simulink model "linear_system"  (R2024b)
settings: Solver=VariableStepAuto  StartTime=0.0  StopTime=10  RelTol=1e-3
values from neighbouring files (symbols this model uses):
  A = double(A_matrix)    [Modelling_AB_Matrix_Calculation.m]
  B = double(B_matrix)    [Modelling_AB_Matrix_Calculation.m]
  C = eye(size(A))    [Modelling_AB_Matrix_Calculation.m]
  config = [l_f, l_r, l_b, l_l]    [Modelling_AB_Matrix_Calculation.m]    (also in Non_linear_trim_solver.m = configs(i, :))
  K = [-0.1 2.30105727721e-17 0.1 -1.6517764485e-17 2.5369137881e-16 -0.1 7.90565190817e-17 0.1 0.158113883008 0.158113883008 0.158113883008 0.158113883008 ... (48 elements, 4x12)]    [K_reference.mat]
libraries: uavutilslib x3
settings Model: Creator=kaleb  LastModifiedBy=kaleb

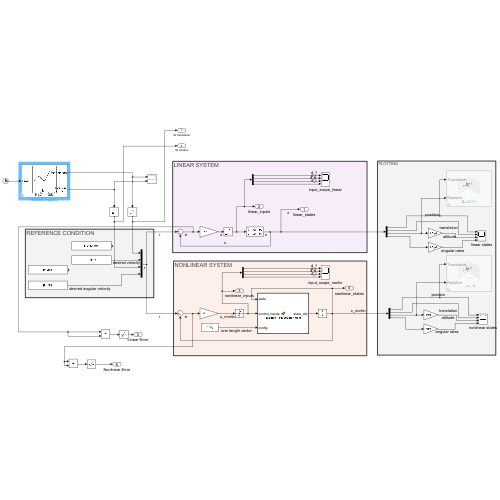
[thumbnail: Simulink's stored preview of the top-level diagram]
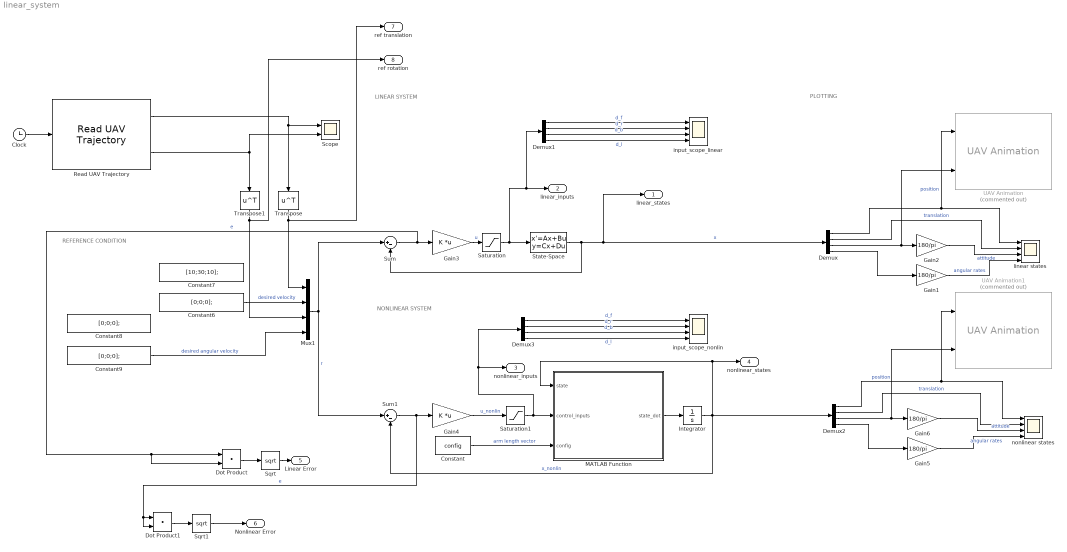
== system linear_system ==
  note: PLOTTING
  note: REFERENCE CONDITION
  note: LINEAR SYSTEM
  note: NONLINEAR SYSTEM
  Clock : Clock
  Constant : Constant  Value=config  OutDataTypeStr=Inherit: Inherit via back propagation
  Constant6 : Constant  Value=[0;0;0];  SampleTime=1/50
  Constant7 : Constant  Value=[10;30;10];  SampleTime=1/50
  Constant8 : Constant  Value=[0;0;0];  SampleTime=1/50
  Constant9 : Constant  Value=[0;0;0];  SampleTime=1/50
  Demux{,1..3} (4 alike) : Demux
  Dot Product : DotProduct  OutDataTypeStr=Inherit: Inherit via internal rule
  Dot Product1 : DotProduct  OutDataTypeStr=Inherit: Inherit via internal rule
  Gain{1..2,5..6} (4 alike) : Gain  Gain=180/pi
  Gain3 : Gain  Gain=K  Multiplication=Matrix(K*u)
  Gain4 : Gain  Gain=K  Multiplication=Matrix(K*u)
  Integrator : Integrator  InitialCondition=[0,0,0 ,5,0,0 ,0,-pi/4,0 ,0,0,0]'
  MATLAB Function : MATLAB Function  TreatAsAtomicUnit=on
  Mux1 : Mux
  Read UAV Trajectory : uavutilslib/Read UAV Trajectory  TrajectorySource=From trajectory object in workspace  ScenarioObj=singleUAVScenario  PlatformName=UAV  TrajectoryObj=T  TransformToENU=off  FrameConversionDisplay=NED → NED
  Saturation : Saturate  UpperLimit=10  LowerLimit=-10
  Saturation1 : Saturate  UpperLimit=20  LowerLimit=-20
  Scope : Scope  NumInputPorts=2
  Sqrt : Sqrt
  Sqrt1 : Sqrt
  State-Space : StateSpace  A=A  B=B  C=C  D=zeros(12,4)  InitialCondition=[0,0,0, 5,0,0, 0,-pi/4,0, 0,0,0];  ContinuousStateAttributes={'pn','pe','h','u','v','w','phi','theta','psi','p','q','r'}
  Sum : Sum  Inputs=|+-
  Sum1 : Sum  Inputs=|+-
  Transpose : Math  Operator=transpose
  Transpose1 : Math  Operator=transpose
  UAV Animation : uavutilslib/UAV Animation  Commented=on  NumUAV=1  DynamicUAVConfig=off  UAVType=Multirotor  UAVSize=0.5  UAVColor=[0.5 0.5 0.5]  UAVTrajectoryAlpha=1  InertialZDirection=Down  RotationFormat=Euler ZYX  DrawMarkers=off  SampleTime=0.1
  UAV Animation1 : uavutilslib/UAV Animation  Commented=on  NumUAV=1  DynamicUAVConfig=off  UAVType=Multirotor  UAVSize=0.5  UAVColor=[0.5 0.5 0.5]  UAVTrajectoryAlpha=1  InertialZDirection=Down  RotationFormat=Euler ZYX  DrawMarkers=off  SampleTime=0.1
  input_scope_linear : Scope  NumInputPorts=4
  input_scope_nonlin : Scope  NumInputPorts=4
  linear states : Scope  NumInputPorts=4
  nonlinear states : Scope  NumInputPorts=4
  linear_states : Outport
  linear_inputs : Outport  Port=2
  nonlinear_inputs : Outport  Port=3
  nonlinear_states : Outport  Port=4
  Linear Error : Outport  Port=5
  Nonlinear Error : Outport  Port=6
  ref translation : Outport  Port=7
  ref rotation : Outport  Port=8
  wires:
  State-Space/1 -> linear_states/1, Demux/1, Sum/2  "x"
  Demux1/1 -> input_scope_linear/1  "d_f"
  Demux1/2 -> input_scope_linear/2  "d_r"
  Demux1/3 -> input_scope_linear/3  "d_b"
  Demux1/4 -> input_scope_linear/4  "d_l"
  Gain3/1 -> Saturation/1  "u"
  Sum/1 -> Gain3/1, Dot Product/1, Dot Product/2  "e"
  Gain4/1 -> Saturation1/1  "u_nonlin"
  Constant/1 -> MATLAB Function/3(config)  "arm length vector"
  Integrator/1 -> Sum1/2, Demux2/1, MATLAB Function/1(state), nonlinear_states/1  "x_nonlin"
  MATLAB Function/1(state_dot) -> Integrator/1
  Sum1/1 -> Gain4/1, Dot Product1/1, Dot Product1/2  "e"
  Demux2/1 -> nonlinear states/1, UAV Animation1/1  "position"
  Demux2/2 -> nonlinear states/2  "translation"
  Demux2/3 -> Gain6/1, UAV Animation1/2
  Demux2/4 -> Gain5/1
  Gain5/1 -> nonlinear states/4  "angular rates"
  Gain6/1 -> nonlinear states/3  "attitude"
  Demux/2 -> linear states/2  "translation"
  Gain2/1 -> linear states/3  "attitude"
  Demux/1 -> linear states/1, UAV Animation/1  "position"
  Gain1/1 -> linear states/4  "angular rates"
  Demux/4 -> Gain1/1
  Demux/3 -> UAV Animation/2, Gain2/1
  Demux3/2 -> input_scope_nonlin/2  "d_r"
  Demux3/3 -> input_scope_nonlin/3  "d_b"
  Demux3/1 -> input_scope_nonlin/1  "d_f"
  Demux3/4 -> input_scope_nonlin/4  "d_l"
  Constant9/1 -> Mux1/4  "desired angular velocity"
  Constant6/1 -> Mux1/2  "desired velocity"
  Mux1/1 -> Sum/1, Sum1/1  "r"
  Sqrt/1 -> Linear Error/1
  Dot Product/1 -> Sqrt/1
  Sqrt1/1 -> Nonlinear Error/1
  Dot Product1/1 -> Sqrt1/1
  Saturation1/1 -> Demux3/1, nonlinear_inputs/1, MATLAB Function/2(control_inputs)
  Saturation/1 -> Demux1/1, linear_inputs/1, State-Space/1
  Clock/1 -> Read UAV Trajectory/1
  Read UAV Trajectory/1 -> Transpose/1, Scope/1
  Read UAV Trajectory/2 -> Scope/2, Transpose1/1
  Transpose/1 -> Mux1/1, ref translation/1
  Transpose1/1 -> ref rotation/1, Mux1/3

== matlab function linear_system/MATLAB Function ==
  data: state input; control_inputs input; config input; state_dot output
%% Equation of motion calculation
function state_dot = calculate_quadcopter_eom(state, control_inputs, config)

l_f = config(1);
l_r = config(2);
l_b = config(3);
l_l = config(4);

% state_dot = zeros(12, 1);

t_motor = 31/1000;   % Motor thickness (m)
t_prop = 2/1000;    % Propeller thickness (m)
d_cube = 0.10;    % Cube dimension (m)
m_motor = 58/1000;   % Motor mass (kg)
m_prop = 21/1000;    % Propeller mass (kg)
m_arm = 65/1000;     % Arm mass (kg)
m_cube = 0.69;    % Cube mass (kg)
r_motor = 28/1000;   % Motor radius (m)
r_prop = 25.4/100;    % Propeller radius (m)

g = 9.81; % Gravity (kg/m^2)
k1 = 1;   % Thrust coefficient
k2 = 0.2; % Torque coefficient

[CG_matrix, J_matrix_body, m_tot] = calculate_CG_Moment_of_inertia(config);

X_cg = CG_matrix(1);
Y_cg = CG_matrix(2);

% Function to calculate the equations of motion of the quadcopter
% Inputs:
%   state: [pn; pe; h; u; v; w; phi; theta; psi; p; q; r]
%   control_inputs: [delta_f; delta_r; delta_b; delta_l]
%   J_matrix_body: Moment of inertia matrix [Jx, Jy, Jz]
%   m_tot: Total mass of the quadcopter
%   k1: Thrust coefficient
%   k2: Torque coefficient
%   g: Gravitational acceleration
%   l_f, l_r, l_b, l_l: Individual arm lengths for front, right, back, and left rotors
% Outputs:
%   state_dot: Time derivatives of the state vector
% load_constant_values

% Extract state variables
pn = state(1); pe = state(2); h = state(3);
u = state(4); v = state(5); w = state(6);
phi = state(7); theta = state(8); psi = state(9);
p = state(10); q = state(11); r = state(12);
% 
% Extract control inputs
delta_f = control_inputs(1);
delta_r = control_inputs(2);
delta_b = control_inputs(3);
delta_l = control_inputs(4);

% Position Dynamics
position_matrix = [
    cos(theta)*cos(psi), sin(phi)*sin(theta)*cos(psi) - cos(phi)*sin(psi), cos(phi)*sin(theta)*cos(psi) + sin(phi)*sin(psi);
    cos(theta)*sin(psi), sin(phi)*sin(theta)*sin(psi) + cos(phi)*cos(psi), cos(phi)*sin(theta)*sin(psi) - sin(phi)*cos(psi);
    sin(theta), -sin(phi)*cos(theta), -cos(phi)*cos(theta)
    ];
position_vector = [u; v; w];
position_dot = position_matrix * position_vector;

% Linear Velocity Dynamics
linear_velocity_matrix = [
    0, r, -q;
    -r, 0, p;
    q, -p, 0
    ];
gravity_vector = [-g*sin(theta); g*cos(theta)*sin(phi); g*cos(theta)*cos(phi)];
control_force = [0; 0; -k1 * (delta_f + delta_r + delta_b + delta_l) / m_tot];
linear_velocity_dot = linear_velocity_matrix * [u; v; w] + gravity_vector + control_force;

% Angular Velocity Dynamics
angular_velocity_matrix = [
    1, sin(phi)*tan(theta), cos(phi)*tan(theta);
    0, cos(phi), -sin(phi);
    0, sin(phi)/cos(theta), cos(phi)/cos(theta)
    ];
angular_velocity_dot = angular_velocity_matrix * [p; q; r];

% Rotational Dynamics
% Torques due to rotor thrusts
tau_x = - (l_r-Y_cg) * k1 * delta_r - (l_l-Y_cg) * k1 * delta_l; % Front-back torques
tau_y = (l_f-X_cg) * k1 * delta_f + (l_b-X_cg) * k1 * delta_b; % Right-left torques
tau_z = k2 * (-delta_f + delta_r - delta_b + delta_l); % Yaw torque due to rotor drag

% Total torques
control_torque = [tau_x; tau_y; tau_z];

% Gyroscopic effects
rotational_dynamics_matrix = [
    (J_matrix_body(2, 2) - J_matrix_body(3, 3)) / J_matrix_body(1, 1), 0, 0;
    0, (J_matrix_body(3, 3) - J_matrix_body(1, 1)) / J_matrix_body(2, 2), 0;
    0, 0, (J_matrix_body(1, 1) - J_matrix_body(2, 2)) / J_matrix_body(3, 3)
    ];
rotational_coupling = [q * r; p * r; p * q];
rotational_velocity_dot = rotational_dynamics_matrix * rotational_coupling + (J_matrix_body \ control_torque);
rotational_velocity_dot = inv(J_matrix_body) * (control_torque - cross([p;q;r], J_matrix_body*[p;q;r]));


% Combine EOMs
state_dot = [position_dot; linear_velocity_dot; angular_velocity_dot; rotational_velocity_dot];
end
